simulink model "HandlingTest"  (R2022a)
settings: Solver=ode5  StartTime=0.0  StopTime=inf  RelTol=1e-3
values from neighbouring files (symbols this model uses):
  simulinkStructInitial = simulinkStruct.signals.values(1,:)    [setupHandlingTest.m]
undefined symbols (not defined in the file or in its folder): opts, Serial_Port, Standard_Devices, UDP_Protocol
libraries: sldrtlib x3, sharedtransform x1
settings Model: Creator=Simonas  LastModifiedBy=sudo
settings HardwareCC: ProdBitPerLong=64  ProdHWDeviceType=Intel->x86-64 (Linux 64)
settings RTWCC: Description=Simulink Desktop Real-Time  SystemTargetFile=sldrt.tlc  TemplateMakefile=sldrt.tmf  RTWCompilerOptimization=on
settings CodeAppCC: MaxIdLength=95
settings SimulinkDesktopRealTimeCC: TargetLibSuffix=_sldrt.a  TargetPreCompLibLocation=C:\Program Files\MATLAB\R2022a\toolbox\sldrt\lib\win64

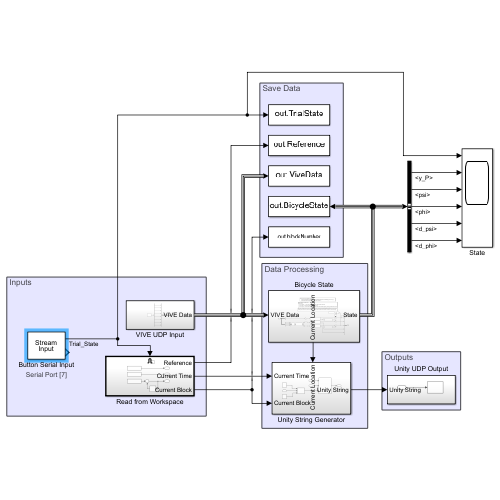
[thumbnail: Simulink's stored preview of the top-level diagram]
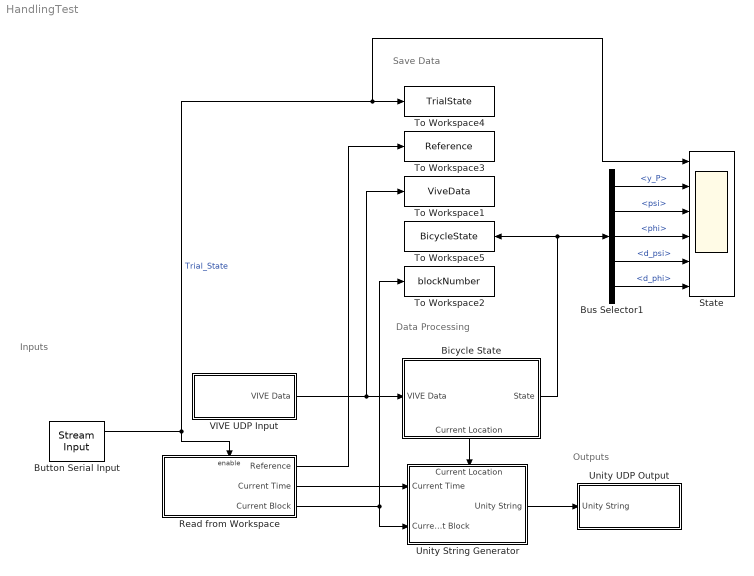
== system HandlingTest ==
  note: Save Data
  note: Inputs
  note: Outputs
  note: Data Processing
  Bicycle State : Subsystem
      settings: PortSchema="{\"entries\":[{\"content\":{\"sides\":[{\"content\":{\"connectorIds\":[\"In1\"]},\"type\":\"ConnectorPlacement.EquallySpacedRectSide\",\"uuid\":\"c5d89f74-e35e-400b-a49a-6a7c3bbb3cee\"},{\"content\":{\"connectorIds\":[\"Out1\"],\"side\":\"RIGHT\"},\"type\":\"ConnectorPlacement.EquallySpacedRectSide\",\"uuid\":\"d3946c1d-493c-4283-9feb-9c130facb0a9\"},{\"content\":{\"connectorIds\":[],\"side\":\"TOP\"},\"type\":\"ConnectorPlacement.EquallySpacedRectSide\",\"uuid\":\"f7eeef6e-15d0-4138-b893-66df70237323\"},{\"content\":{\"connectorIds\":[\"Out2\"],\"side\":\"BOTTOM\"},\"type\":\"ConnectorPlacement.EquallySpacedRectSide\",\"uuid\":\"d8cc5cfa-3fb7-476d-9b2c-860b356f327e\"}]},\"type\":\"ConnectorPlacement.EquallySpacedConnector\",\"uuid\":\"85360968-76db-44cc-98f9-7355ff2a9269\"}],\"packageUris\":[\"http://schema.mathworks.com/mf0/Connector/R2020b\"],\"version\":\"1.0\"}"
  Bus Selector1 : BusSelector  OutputSignals=y_P,psi,phi,d_psi,d_phi
  Button Serial Input : sldrtlib/Stream Input  SampleTime=opts.T_ser  MaxMissedTicks=1000000  ShowMissedTicks=off  YieldWhenWaiting=off  DrvName=Standard_Devices/Serial_Port  DrvAddress=7  DrvOptions=[9600 8 0 0 0 0 0 0]  DataTypes='int32'  FormatString='%d'  Terminator={'\n', '\r'}  ShowReady=on  ShowError=off
      settings: AttributesFormatString=Serial Port [7]  SourceProductBaseCode=WT
  Read from Workspace : Subsystem  TreatAsAtomicUnit=on
  State : Scope  NumInputPorts=6
  To Workspace1 : ToWorkspace  VariableName=ViveData  SaveFormat=Timeseries  SampleTime=-1
  To Workspace2 : ToWorkspace  VariableName=blockNumber  SaveFormat=Timeseries  SampleTime=-1
  To Workspace3 : ToWorkspace  VariableName=Reference  SaveFormat=Timeseries  SampleTime=-1
  To Workspace4 : ToWorkspace  VariableName=TrialState  SaveFormat=Timeseries  SampleTime=-1
  To Workspace5 : ToWorkspace  VariableName=BicycleState  SaveFormat=Timeseries  SampleTime=-1
  Unity String Generator : Subsystem
      settings: PortSchema="{\"entries\":[{\"content\":{\"sides\":[{\"content\":{\"connectorIds\":[\"In1\",\"In2\"]},\"type\":\"ConnectorPlacement.EquallySpacedRectSide\",\"uuid\":\"995dcb62-78f8-423c-99d5-aa9c538d86ef\"},{\"content\":{\"connectorIds\":[\"Out1\"],\"side\":\"RIGHT\"},\"type\":\"ConnectorPlacement.EquallySpacedRectSide\",\"uuid\":\"d6e446ff-77b4-4bca-8c68-e505a29969fe\"},{\"content\":{\"connectorIds\":[\"In3\"],\"side\":\"TOP\"},\"type\":\"ConnectorPlacement.EquallySpacedRectSide\",\"uuid\":\"a2ee3f9a-5385-4b4c-abf0-7e00a59d14cf\"}]},\"type\":\"ConnectorPlacement.EquallySpacedConnector\",\"uuid\":\"6b026230-ac01-4f6d-82d7-753dc9fb2975\"}],\"packageUris\":[\"http://schema.mathworks.com/mf0/Connector/R2020b\"],\"version\":\"1.0\"}"
  Unity UDP Output : Subsystem
  VIVE UDP Input : Subsystem
  wires:
  Read from Workspace/3(Current Block) -> Unity String Generator/2(Current Block), To Workspace2/1
  Bus Selector1/1 -> State/2  "<y_P>"
  Bus Selector1/3 -> State/4  "<phi>"
  Bus Selector1/5 -> State/6  "<d_phi>"
  Bus Selector1/4 -> State/5  "<d_psi>"
  Bus Selector1/2 -> State/3  "<psi>"
  Read from Workspace/2(Current Time) -> Unity String Generator/1(Current Time)
  Read from Workspace/1(Reference) -> To Workspace3/1
  VIVE UDP Input/1(VIVE Data) -> Bicycle State/1(VIVE Data), To Workspace1/1
  Bicycle State/2(Current Location) -> Unity String Generator/3(Current Location)
  Bicycle State/1(State) -> Bus Selector1/1, To Workspace5/1
  Button Serial Input/1 -> Read from Workspace/Enable, To Workspace4/1, State/1  "Trial_State"
  Unity String Generator/1(Unity String) -> Unity UDP Output/1(Unity String)

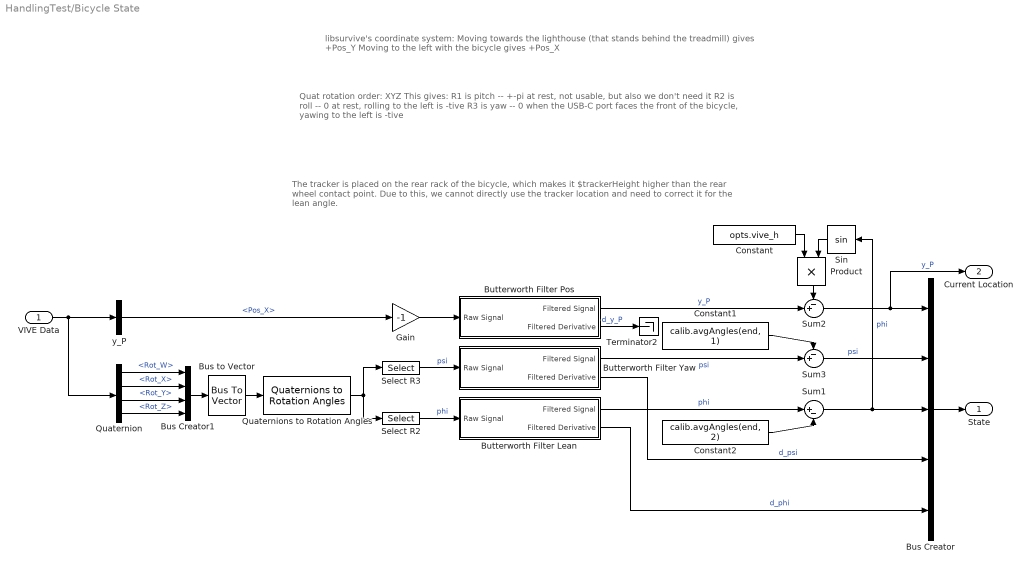
== system HandlingTest/Bicycle State ==
  note: The tracker is placed on the rear rack of the bicycle, which makes it $trackerHeight higher than the rear wheel contact point. Due to this, we cannot directly use the tracker location and need to correct it for the lean angle.
  note: libsurvive's coordinate system:
      | Moving towards the lighthouse (that stands behind the treadmill) gives +Pos_Y
      | Moving to the left with the bicycle gives +Pos_X
  note: Quat rotation order: XYZ
      | This gives:
      | R1 is pitch -- +-pi at rest, not usable, but also we don't need it
      | R2 is roll -- 0 at rest, rolling to the left is -tive
      | R3 is yaw -- 0 when the USB-C port faces the front of the bicycle, yawing to the left is -tive
  VIVE Data : Inport
  Bus Creator : BusCreator  Inputs=5
  Bus Creator1 : BusCreator  Inputs=4
  Bus to Vector : BusToVector
  Butterworth Filter Lean : Subsystem
  Butterworth Filter Pos : Subsystem
  Butterworth Filter Yaw : Subsystem
  Constant : Constant  Value=opts.vive_h
  Constant1 : Constant  Value=calib.avgAngles(end, 1)  SampleTime=opts.T_udp
  Constant2 : Constant  Value=calib.avgAngles(end, 2)  SampleTime=opts.T_udp
  Gain : Gain  Gain=-1
  Product : Product
  Quaternion : BusSelector  OutputSignals=Rot_W,Rot_X,Rot_Y,Rot_Z
  Quaternions to Rotation Angles : sharedtransform/Quaternions to Rotation Angles  rotationOrder=XYZ  aMode=aMode
      settings: SourceProductBaseCode=AE,PW,DR,MT,VE
  Select R2 : Selector  InputPortWidth=3  IndexOptions=Index vector (dialog)  Indices=2  OutputSizes=1
  Select R3 : Selector  InputPortWidth=3  IndexOptions=Index vector (dialog)  Indices=3  OutputSizes=1
  Sin : Trigonometry
  Sum1 : Sum  Inputs=|+-
  Sum2 : Sum  Inputs=-+|
  Sum3 : Sum  Inputs=-+|
  Terminator2 : Terminator
  y_P : BusSelector  OutputSignals=Pos_X
  State : Outport
  Current Location : Outport  Port=2
  wires:
  VIVE Data/1 -> Quaternion/1, y_P/1
  Quaternion/2 -> Bus Creator1/2  "<Rot_X>"
  Quaternion/3 -> Bus Creator1/3  "<Rot_Y>"
  Quaternion/4 -> Bus Creator1/4  "<Rot_Z>"
  Select R2/1 -> Butterworth Filter Lean/1(Raw Signal)  "phi"
  y_P/1 -> Gain/1  "<Pos_X>"
  Bus Creator/1 -> State/1
  Quaternion/1 -> Bus Creator1/1  "<Rot_W>"
  Bus Creator1/1 -> Bus to Vector/1
  Bus to Vector/1 -> Quaternions to Rotation Angles/1
  Quaternions to Rotation Angles/1 -> Select R3/1, Select R2/1
  Gain/1 -> Butterworth Filter Pos/1(Raw Signal)
  Constant/1 -> Product/1
  Sin/1 -> Product/2
  Butterworth Filter Lean/2(Filtered Derivative) -> Bus Creator/5  "d_phi"
  Butterworth Filter Pos/2(Filtered Derivative) -> Terminator2/1  "d_y_P"
  Select R3/1 -> Butterworth Filter Yaw/1(Raw Signal)  "psi"
  Butterworth Filter Yaw/1(Filtered Signal) -> Sum3/2  "psi"
  Butterworth Filter Yaw/2(Filtered Derivative) -> Bus Creator/4  "d_psi"
  Butterworth Filter Pos/1(Filtered Signal) -> Sum2/2  "y_P"
  Sum2/1 -> Current Location/1, Bus Creator/1  "y_P"
  Product/1 -> Sum2/1
  Sum1/1 -> Sin/1, Bus Creator/3  "phi"
  Sum3/1 -> Bus Creator/2  "psi"
  Constant1/1 -> Sum3/1
  Butterworth Filter Lean/1(Filtered Signal) -> Sum1/1  "phi"
  Constant2/1 -> Sum1/2

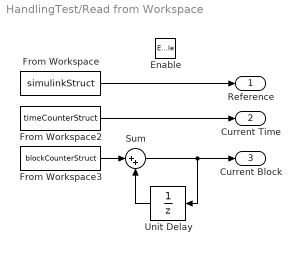
== system HandlingTest/Read from Workspace ==
  Enable : EnablePort  StatesWhenEnabling=reset
  From Workspace : FromWorkspace  VariableName=simulinkStruct  SampleTime=opts.T_ref  Interpolate=off  OutputAfterFinalValue=Cyclic repetition
  From Workspace2 : FromWorkspace  VariableName=timeCounterStruct  SampleTime=opts.T_ref  Interpolate=off  OutputAfterFinalValue=Cyclic repetition
  From Workspace3 : FromWorkspace  VariableName=blockCounterStruct  SampleTime=opts.T_ref  Interpolate=off  OutputAfterFinalValue=Cyclic repetition
  Sum : Sum  Inputs=|++
  Unit Delay : UnitDelay  InitialCondition=1  SampleTime=opts.T_ref  HasFrameUpgradeWarning=on
  Reference : Outport  InitialOutput=simulinkStructInitial
  Current Time : Outport  Port=2  OutputWhenDisabled=reset  InitialOutput=0
  Current Block : Outport  Port=3  OutputWhenDisabled=reset  InitialOutput=1
  wires:
  From Workspace/1 -> Reference/1
  From Workspace2/1 -> Current Time/1
  From Workspace3/1 -> Sum/1
  Sum/1 -> Unit Delay/1, Current Block/1
  Unit Delay/1 -> Sum/2

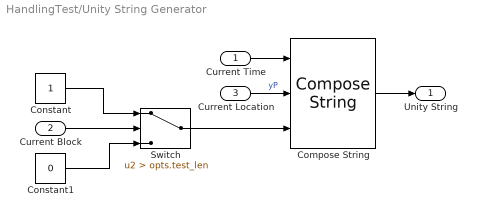
== system HandlingTest/Unity String Generator ==
  Current Time : Inport
  Current Block : Inport  Port=2
  Current Location : Inport  Port=3
  Compose String : ComposeString  Format="\"%.0f,%.3f,%.0f\\n\""
  Constant : Constant
  Constant1 : Constant  Value=0
  Switch : Switch  Criteria=u2 > Threshold  Threshold=opts.test_len  SaturateOnIntegerOverflow=off  InputSameDT=off
  Unity String : Outport  OutDataTypeStr=string
  wires:
  Current Time/1 -> Compose String/1
  Current Location/1 -> Compose String/2  "yP"
  Compose String/1 -> Unity String/1
  Current Block/1 -> Switch/2
  Constant/1 -> Switch/1
  Constant1/1 -> Switch/3
  Switch/1 -> Compose String/3

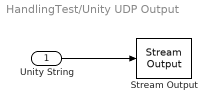
== system HandlingTest/Unity UDP Output ==
  Unity String : Inport
  Stream Output : sldrtlib/Stream Output  SampleTime=opts.T_udp  MaxMissedTicks=1000000  ShowMissedTicks=off  YieldWhenWaiting=on  DrvName=Standard_Devices/UDP_Protocol  DrvAddress=8005  DrvOptions=[0 8006 49 50 55 46 48 46 48 46 49 0 0 0 0 0 0 0 0 0 0 0 0 0 0 0 0 0 0 0 0 0 0 0 0 0 0 0 0 0 0 0 0 0 0 0 0 0 0 0 0 0 0 0 0 0 0 0 0 0 0 0 0 0 0 0 0 0 0 0 0 0 0 0 0 0 0 0 0 0 0 0 0 0 0 0 0 0 0 0 0 0 0 0 0 0 0 0 0 0 0 0 0 0 0 0 0 0 0 0 0 0 0 0 0 0 0 0 0 0 0 0 0 0 0 0 0 0 0 0 0 0 0 0 0 0 0 0 0 0 0 0 0 0 0 0 0 0 0 0 0 0 0 0 0 0 0 0 0 0 0 0 0 0 0 0 0 0 0 0 0 0 0 0 0 0 0 0 0 0 0 0 0 0 0 0 0 0 0 0 0 0 0 0 0 0 0 0 0 0 0 0 0 0 0 0 0 0 0 0 0 0 0 0 0 0 0 0 0 0 0 0 0 0 0 0 0 0 0 0 0 0 0 0 0 0 0 0 0 0 0 0 0 0 0 0 0 0 0 0 0 0 0 0 0 0]  PortSizes=1  FormatString='%s'  ShowReady=off  ShowError=off  InitialValue=[]  FinalValue=[]
      settings: AttributesFormatString=UDP Protocol [8005]  SourceProductBaseCode=WT
  wires:
  Unity String/1 -> Stream Output/1

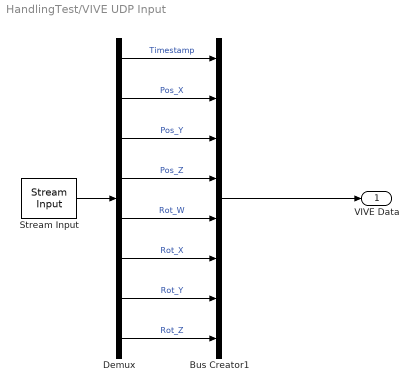
== system HandlingTest/VIVE UDP Input ==
  Bus Creator1 : BusCreator  Inputs=8
  Demux : Demux  Outputs=8
  Stream Input : sldrtlib/Stream Input  SampleTime=opts.T_udp  MaxMissedTicks=1000000  ShowMissedTicks=off  YieldWhenWaiting=on  DrvName=Standard_Devices/UDP_Protocol  DrvAddress=4950  DrvOptions=[0 16385 0 0 0 0 0 0 0 0 0 0 0 0 0 0 0 0 0 0 0 0 0 0 0 0 0 0 0 0 0 0 0 0 0 0 0 0 0 0 0 0 0 0 0 0 0 0 0 0 0 0 0 0 0 0 0 0 0 0 0 0 0 0 0 0 0 0 0 0 0 0 0 0 0 0 0 0 0 0 0 0 0 0 0 0 0 0 0 0 0 0 0 0 0 0 0 0 0 0 0 0 0 0 0 0 0 0 0 0 0 0 0 0 0 0 0 0 0 0 0 0 0 0 0 0 0 0 0 0 0 0 0 0 0 0 0 0 0 0 0 0 0 0 0 0 0 0 0 0 0 0 0 0 0 0 0 0 0 0 0 0 0 0 0 0 0 0 0 0 0 0 0 0 0 0 0 0 0 0 0 0 0 0 0 0 0 0 0 0 0 0 0 0 0 0 0 0 0 0 0 0 0 0 0 0 0 0 0 0 0 0 0 0 0 0 0 0 0 0 0 0 0 0 0 0 0 0 0 0 0 0 0 0 0 0 0 0 0 0 0 0 0 0 0 0 0 0 0 0 0 0 0 0 0 0]  DataTypes={'8*double'}  FormatString='%f,%f,%f,%f,%f,%f,%f,%f'  Terminator='\n'  ShowReady=off  ShowError=off
      settings: AttributesFormatString=UDP Protocol [4950]  SourceProductBaseCode=WT
  VIVE Data : Outport
  wires:
  Demux/4 -> Bus Creator1/4  "Pos_Z"
  Demux/5 -> Bus Creator1/5  "Rot_W"
  Demux/7 -> Bus Creator1/7  "Rot_Y"
  Demux/6 -> Bus Creator1/6  "Rot_X"
  Demux/1 -> Bus Creator1/1  "Timestamp"
  Demux/2 -> Bus Creator1/2  "Pos_X"
  Demux/8 -> Bus Creator1/8  "Rot_Z"
  Demux/3 -> Bus Creator1/3  "Pos_Y"
  Bus Creator1/1 -> VIVE Data/1
  Stream Input/1 -> Demux/1

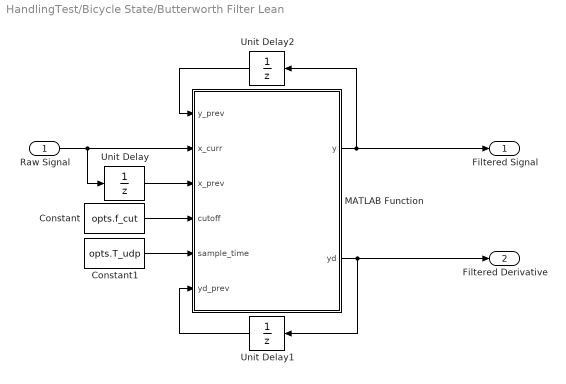
== system HandlingTest/Bicycle State/Butterworth Filter Lean ==
  Raw Signal : Inport
  Constant : Constant  Value=opts.f_cut  SampleTime=opts.T_udp
  Constant1 : Constant  Value=opts.T_udp  SampleTime=opts.T_udp
  MATLAB Function : MATLAB Function  TreatAsAtomicUnit=on
  Unit Delay : UnitDelay  SampleTime=opts.T_udp  HasFrameUpgradeWarning=on
  Unit Delay1 : UnitDelay  SampleTime=opts.T_udp  HasFrameUpgradeWarning=on
  Unit Delay2 : UnitDelay  SampleTime=opts.T_udp  HasFrameUpgradeWarning=on
  Filtered Signal : Outport
  Filtered Derivative : Outport  Port=2
  wires:
  MATLAB Function/1(y) -> Unit Delay2/1, Filtered Signal/1
  MATLAB Function/2(yd) -> Unit Delay1/1, Filtered Derivative/1
  Raw Signal/1 -> Unit Delay/1, MATLAB Function/2(x_curr)
  Unit Delay/1 -> MATLAB Function/3(x_prev)
  Constant/1 -> MATLAB Function/4(cutoff)
  Constant1/1 -> MATLAB Function/5(sample_time)
  Unit Delay2/1 -> MATLAB Function/1(y_prev)
  Unit Delay1/1 -> MATLAB Function/6(yd_prev)

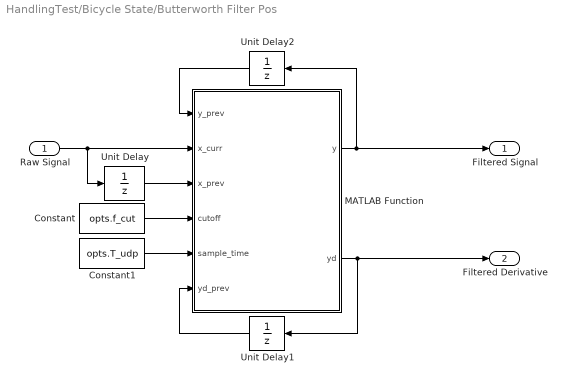
== system HandlingTest/Bicycle State/Butterworth Filter Pos ==
  Raw Signal : Inport
  Constant : Constant  Value=opts.f_cut  SampleTime=opts.T_udp
  Constant1 : Constant  Value=opts.T_udp  SampleTime=opts.T_udp
  MATLAB Function : MATLAB Function  TreatAsAtomicUnit=on
  Unit Delay : UnitDelay  SampleTime=opts.T_udp  HasFrameUpgradeWarning=on
  Unit Delay1 : UnitDelay  SampleTime=opts.T_udp  HasFrameUpgradeWarning=on
  Unit Delay2 : UnitDelay  SampleTime=opts.T_udp  HasFrameUpgradeWarning=on
  Filtered Signal : Outport
  Filtered Derivative : Outport  Port=2
  wires:
  MATLAB Function/1(y) -> Unit Delay2/1, Filtered Signal/1
  MATLAB Function/2(yd) -> Unit Delay1/1, Filtered Derivative/1
  Raw Signal/1 -> Unit Delay/1, MATLAB Function/2(x_curr)
  Unit Delay/1 -> MATLAB Function/3(x_prev)
  Constant/1 -> MATLAB Function/4(cutoff)
  Constant1/1 -> MATLAB Function/5(sample_time)
  Unit Delay2/1 -> MATLAB Function/1(y_prev)
  Unit Delay1/1 -> MATLAB Function/6(yd_prev)

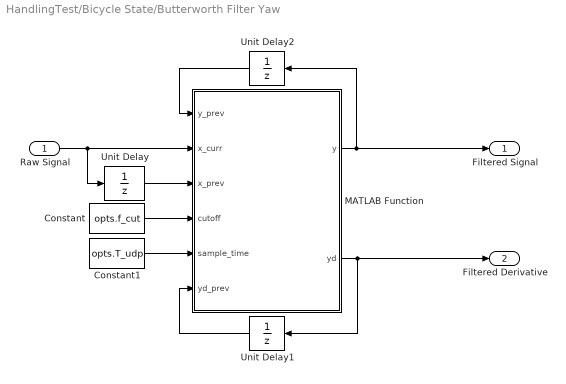
== system HandlingTest/Bicycle State/Butterworth Filter Yaw ==
  Raw Signal : Inport
  Constant : Constant  Value=opts.f_cut  SampleTime=opts.T_udp
  Constant1 : Constant  Value=opts.T_udp  SampleTime=opts.T_udp
  MATLAB Function : MATLAB Function  TreatAsAtomicUnit=on
  Unit Delay : UnitDelay  SampleTime=opts.T_udp  HasFrameUpgradeWarning=on
  Unit Delay1 : UnitDelay  SampleTime=opts.T_udp  HasFrameUpgradeWarning=on
  Unit Delay2 : UnitDelay  SampleTime=opts.T_udp  HasFrameUpgradeWarning=on
  Filtered Signal : Outport
  Filtered Derivative : Outport  Port=2
  wires:
  MATLAB Function/1(y) -> Unit Delay2/1, Filtered Signal/1
  MATLAB Function/2(yd) -> Unit Delay1/1, Filtered Derivative/1
  Raw Signal/1 -> Unit Delay/1, MATLAB Function/2(x_curr)
  Unit Delay/1 -> MATLAB Function/3(x_prev)
  Constant/1 -> MATLAB Function/4(cutoff)
  Constant1/1 -> MATLAB Function/5(sample_time)
  Unit Delay2/1 -> MATLAB Function/1(y_prev)
  Unit Delay1/1 -> MATLAB Function/6(yd_prev)

== matlab function HandlingTest/Bicycle State/Butterworth Filter Lean/MATLAB Function ==
  data: y_prev input; y output; x_curr input; x_prev input; cutoff input; sample_time input; yd_prev input; yd output
function [y, yd] = realtime_filter(y_prev, x_curr, x_prev, ...
                                   cutoff, sample_time, yd_prev)
a = (2*pi * cutoff^2);
b = sqrt(2) * 2*pi * cutoff;
h = sample_time;
denom = 4 + 2*h*b + h^2*a;

A = (4 + 2*h*b - h^2*a) / denom;
B = 4*h / denom;
C = -4*h*a / denom;
D = (4 - 2*h*b - h^2*a) / denom;
E = 2*h^2*a / denom;
F = 4*h*a / denom;

y = A * y_prev + B * yd_prev + E * (x_curr + x_prev) / 2;
yd = C * y_prev + D * yd_prev + F * (x_curr + x_prev) / 2;

== matlab function HandlingTest/Bicycle State/Butterworth Filter Pos/MATLAB Function ==
  data: y_prev input; y output; x_curr input; x_prev input; cutoff input; sample_time input; yd_prev input; yd output
function [y, yd] = realtime_filter(y_prev, x_curr, x_prev, ...
                                   cutoff, sample_time, yd_prev)
a = (2*pi * cutoff^2);
b = sqrt(2) * 2*pi * cutoff;
h = sample_time;
denom = 4 + 2*h*b + h^2*a;

A = (4 + 2*h*b - h^2*a) / denom;
B = 4*h / denom;
C = -4*h*a / denom;
D = (4 - 2*h*b - h^2*a) / denom;
E = 2*h^2*a / denom;
F = 4*h*a / denom;

y = A * y_prev + B * yd_prev + E * (x_curr + x_prev) / 2;
yd = C * y_prev + D * yd_prev + F * (x_curr + x_prev) / 2;

== matlab function HandlingTest/Bicycle State/Butterworth Filter Yaw/MATLAB Function ==
  data: y_prev input; y output; x_curr input; x_prev input; cutoff input; sample_time input; yd_prev input; yd output
function [y, yd] = realtime_filter(y_prev, x_curr, x_prev, ...
                                   cutoff, sample_time, yd_prev)
a = (2*pi * cutoff^2);
b = sqrt(2) * 2*pi * cutoff;
h = sample_time;
denom = 4 + 2*h*b + h^2*a;

A = (4 + 2*h*b - h^2*a) / denom;
B = 4*h / denom;
C = -4*h*a / denom;
D = (4 - 2*h*b - h^2*a) / denom;
E = 2*h^2*a / denom;
F = 4*h*a / denom;

y = A * y_prev + B * yd_prev + E * (x_curr + x_prev) / 2;
yd = C * y_prev + D * yd_prev + F * (x_curr + x_prev) / 2;
